simulink library "carnot"  (R2018b)
settings: Solver=VariableStepAuto  StartTime=0.0  StopTime=10.0  RelTol=1e-3
undefined symbols (not defined in the file or in its folder): A, A_earth, acol, Acol, ActPower1, ActPower2, ActPower3, Ad, Ad0, Ar, Au, Au0, Azimuth_Angle, B, Bd, Bd0, Br, Bu, Bu0, C, c1, c2, c3, c33, c4, c5, c6, CarnotCallbacks_Density, CarnotCallbacks_Enthalpy, CarnotCallbacks_Enthalpy2Temperature, CarnotCallbacks_Entropy, CarnotCallbacks_Evaporation_Enthalpy, CarnotCallbacks_GlobalMessageLevel, CarnotCallbacks_Grashof, CarnotCallbacks_Heat_Capacity, CarnotCallbacks_Kinematic_Viscosity, CarnotCallbacks_PMV_PPD, CarnotCallbacks_Prandtl, CarnotCallbacks_Saturation_Property, CarnotCallbacks_Saturation_Temperature, CarnotCallbacks_Saturation_Value_Water, CarnotCallbacks_Specific_Volume, CarnotCallbacks_Thermal_Conductivity, CarnotCallbacks_Vapour_Content, CarnotCallbacks_Vapour_Pressure, Cd, Cdl, Cr, Cu, Davies, Dd, DE_TRY2010_04_averageYear, delta_grd, density, DiameterLastPiece, dl, DPConstant, DPLinear, DPQuadratic, Dr ... (+59)
libraries: $bdroot x429, simulink x36, simulink_extras x12
(part 10 of 22)

== system carnot/Source/Solar_Thermal ==
  Collector_1xN : Subsystem  mask(collector 1xN){acol=2.3, len=2, eta0=0.8, u1=3.5, u2=0.02, u3=0, uwind=0, c_col=1e4, lin=10, qua=10, tini=20, nodes=5}
      mask prompts: acol "collector surface (aperture) in [m²]"; len "length between inlet and outlet [m]"; eta0 "optical efficiency [-]"; u1 "linear heat loss coefficient [W/(m²*K)]"; u2 "quadratic heat loss coefficient [W/(m*K)²]"; u3 "radiative loss coefficient [W/(m²*K)]"; uwind "wind dependent heat loss [W/(m²*K*m/s)]"; c_col "effective heat capacity of collector [J/(m²*K)]"; lin "linear pressure drop Pa/(kg/s)"; qua "quadratic  pressure drop Pa/(kg/s)²"; tini "initial temperature [degree Celsius]"; nodes "number of nodes"
      mask help:
      | Model for tested collectors. Enter test results in this mask.
      | Look under mask to change the incidence angle modifier, the pressure drop and the radiation calculation method.
      mask init:
      | acol = max(acol, 0.01);
      | eta0 = max(eta0,0);
      | c_col = max(c_col, 0.1);
      mask Help: web(fullfile(path_carnot('help'),'Collector_1xN.html'),'-helpbrowser')
      mask DialogControl ParameterTabVar0 Prompt: Geometry
      mask DialogControl ParameterTabVar01 Prompt: Coll.Parameters
      mask DialogControl ParameterTabVar012 Prompt: Hydraulic
      mask DialogControl ParameterTabVar0123 Prompt: Calculation
      mask Display: plot(-10,0,80,78,[10 16 66 60 10],[16 10 60 66 16],[8,13],[8,13],[63,68],[63,68])
  Collector_Unglazed : Subsystem  mask(Unglazed solar thermal collector){tini=0.1, Ncollector=1, PathName=fullfile(path_carnot('libsl'), 'Source', 'Solar_Thermal', 'Collector_Unglazed', 'parameter_set'), FileName='DefaultCollectorUnglazed.mat', userPath=off, userParam=off, acol=2.544, len=2.1, nodes=10, fta=0.9, eps=0.9, u0l=40, u0c=1, u0g=40, u1l=8, u1c=1, u1g=8, u1e=0.01, hi=200, capa=5000, capf=4000, SensorTimeConstant=10, dplin=5504.4, dpqua=6222.096}
      mask prompts: tini "Initial temperature [°C]"; Ncollector "Number of collectors in parallel"; PathName "Path"; FileName "Parameter set"; userPath "Edit path and name of parameter set"; userParam "User defined parameters"; acol "Collector surface (aperture) in [m²]"; len "Length between inlet and outlet [m]"; nodes "Number of nodes (>=2)"; fta "Absorption coefficient of the absorber [-]"; eps "Thermal emissivity of the absorber (0..1)"; u0l "U0L heat transfer for losses [W/(m²*K)]"; u0c "U0C heat transfer for condensation [W/(m²*K)]"; u0g "U0G heat transfer for gains [W/(m²*K)]"; u1l "U1L wind dependent heat transfer for losses [W/(m²*K*m/s)]"; u1c "U1C wind dependent heat transfer for condensation [W/(m²*K*m/s)]"; u1g "U1G wind dependent heat transfer for gains [W/(m²*K*m/s)]"; u1e "U1E wind dependancy of optical efficiency in W/(m²*m/s)"; hi "HI heat transfer between collector and tube [W/(m²*K)]"; capa "Effective heat capacity of absorber [J/(m²*K)]"; capf "Effective heat capacity of fluid [J/(m²*K)]"; SensorTimeConstant "Time constant of temperature sensor [s]"; dplin "Linear pressure drop in Pa/(kg/s)"; dpqua "Quadratic pressure drop in Pa/(kg/s)²"
      mask help:
      | 2xN node model for an unglazed solar thermal collectors including condensation effects for temperatures below dewpoint.
      | c_abs*dTp/dt=qdot_solar-qdot_conv_gain-qdot_conv_loss-qdot_cond -qdot_sky-qdot_fluid
      | qdot_solar = absorbed_solar_radiation - U1E*Iglb*vwind
      | qdot_conv_gain = fconv * (U0G + U1G*vwind)*(Tp - Tamb)
      | qdot_conv_loss = (1-fconv)*(U0L + U1L*vwind)*(Tp - Tamb)
      | qdot_cond = fcond*(U0C + U1C*vwind)*ccond*(ps(Tdew) - ps(Tp))
      | qdot_sky = e * const_sigma*((Tp+273)^4 - (Tsky+273)^4)
      | qdot_fluid = HI*(Tp-Tfluid)
      | fconv = 1 if Tp > Tamb, 0 otherwise
      | fcond = 1 if Tp below dewpoint, 0 otherwise
      mask init:
      | [ok, param] = CarnotCallbacks_CollectorUnglazedConf('SetParameters',gcbh,PathName,FileName);
      mask Help: web(fullfile(path_carnot('help'),'Collector_Unglazed.html'),'-helpbrowser')
      mask TypeOptions tini: Collector_Unglazed/tini | T_Sensor1/t0
      mask TypeOptions Ncollector: Ncollector/Value | Gain/Gain | Gain3/Gain
      mask Callback userPath: [ok, param] = CarnotCallbacks_CollectorUnglazedConf('UserEdit',gcbh);
      mask Callback userParam: [ok, param] = CarnotCallbacks_CollectorUnglazedConf('UserEdit',gcbh);
      mask TypeOptions acol: Collector_Unglazed/acol
      mask TypeOptions len: Collector_Unglazed/len
      mask TypeOptions nodes: Collector_Unglazed/nodes
      mask TypeOptions fta: Collector_Unglazed/fta
      mask TypeOptions eps: Collector_Unglazed/e_sky
      mask TypeOptions u0l: Collector_Unglazed/uc0loss
      mask TypeOptions u0c: Collector_Unglazed/uc0
      mask TypeOptions u0g: Collector_Unglazed/uc0gain
      mask TypeOptions u1l: Collector_Unglazed/uc1loss
      mask TypeOptions u1c: Collector_Unglazed/uc1
      mask TypeOptions u1g: Collector_Unglazed/uc1gain
      mask TypeOptions u1e: Collector_Unglazed/uc1eta0
      mask TypeOptions hi: Collector_Unglazed/hi
      mask TypeOptions capa: Collector_Unglazed/c_abs
      mask TypeOptions capf: Collector_Unglazed/c_fl
      mask TypeOptions SensorTimeConstant: T_Sensor1/tc
      mask TypeOptions dplin: Collector_Unglazed/lin
      mask TypeOptions dpqua: Collector_Unglazed/qua
      mask DialogControl Container7 Prompt: Calculation
      mask DialogControl ParameterGroupVar Prompt: Picking a parameter set
      mask DialogControl Control3 Prompt: Carnot public data
      mask DialogControl Control3 Callback: [ok, file] = CarnotCallbacks_CollectorUnglazedConf('GetFilename',gcbh, 'public');
      mask DialogControl Control4 Prompt: Carnot internal data
      mask DialogControl Control4 Callback: [ok, file] = CarnotCallbacks_CollectorUnglazedConf('GetFilename',gcbh, 'internal');
      mask DialogControl Control2 Prompt: Selected path
      mask DialogControl Control2 Callback: [ok, file] = CarnotCallbacks_CollectorUnglazedConf('GetFilename',gcbh, 'selected');
      mask DialogControl Container9 Prompt: Parameter values
      mask DialogControl Container8 Prompt: Geometry
      mask DialogControl Container11 Prompt: Thermal
      mask DialogControl Container12 Prompt: Hydraulic
      mask DialogControl Control6 Prompt: Save in Carnot internal data
      mask DialogControl Control6 Callback: [ok, param] = CarnotCallbacks_CollectorUnglazedConf('SaveFilename',gcbh, 'internal','USTC');
      mask DialogControl Control5 Prompt: Save in selected path
      mask DialogControl Control5 Callback: [ok, param] = CarnotCallbacks_CollectorUnglazedConf('SaveFilename',gcbh, 'selected','USTC');
      mask Display:
      | % user defined picture file
      | picfile = fullfile(path_carnot('intlibsl'), ...
      |     'Source','Solar_Thermal','Collector_Unglazed','parameter_set', ...
      |      'Collector_CONF.jpg');
      | 
      | pic = false;
      | 
      | % show internal picture if defined
      | if ~BlockIsInCarnotLibrary    % if not located in library any more
      |     if exist(picfile)
      |         image(imread(picfile), [0.2, 0, 0.7, 1])
      |         set_param(gcb, 'BackgroundColor', 'White')
      |         pic = true;
      |     end
      | end
      | 
      | if ~pic % show public picture
      |     plot([0,70,70,0,0]/140+0.1,         [-0,-0,5,5,-0]/140+0.2, ...
      |         [30,30,100,100,30]/140+0.1,     [100,94,94,100,100]/140+0.2, ...
      |         [32,1]/140+0.1,                 [94,5]/140+0.2, ...
      |         [40,10]/140+0.1,                [94,5]/140+0.2, ...
      |         [49,19]/140+0.1,                [94,5]/140+0.2, ...
      |         [57,27]/140+0.1,                [94,5]/140+0.2, ...
      |         [65,35]/140+0.1,                [94,5]/140+0.2, ...
      |         [73,43]/140+0.1,                [94,5]/140+0.2, ...
      |         [82,51]/140+0.1,                [94,5]/140+0.2, ...
      |         [90,60]/140+0.1,                [94,5]/140+0.2,...
      |         [98,68]/140+0.1,                [94,5]/140+0.2)
      |     set_param(gcb, 'BackgroundColor', 'Yellow')
      | end
  Collector_Unglazed_ISO9806 : Subsystem  mask(Unglazed solar thermal collector){tini=1, Ncollector=2, PathName='current', FileName='Viessmann_SLK_ISO9806_lowCp.mat', userPath=off, userParam=off, acol=2.544, len=2.1, eta0=0.702, bu=0.066, b1=32.64, b2=3.59, c_abs=2*3900, dplin=5504.4, dpqua=6222.096}
      mask prompts: tini "Initial temperature [°C]"; Ncollector "Number of collectors in parallel"; PathName "Path"; FileName "Parameter set"; userPath "Edit path and name of parameter set"; userParam "User defined parameters"; acol "Collector surface (aperture) in [m²]"; len "Length between inlet and outlet [m]"; eta0 "Optical efficiency Eta0 [-]"; bu "bu: wind dependancy of optical efficiency in W/(m²*m/s)"; b1 "b1: heat transfer for losses [W/(m²*K)]"; b2 "b2: wind dependent heat transfer for losses [W/(m²*K*m/s)]"; c_abs "Effective heat capacity of absorber [J/(m²*K)]"; dplin "Linear pressure drop in Pa/(kg/s)"; dpqua "Quadratic pressure drop in Pa/(kg/s)²"
      mask help:
      | ISO 9806 model of an unglazed solar thermal collector.
      |  Qdot = A*G*(eta0*(1-bu*vwind) - (b1 + b2*vwind)*(Tm-Tamb)/G)
      |  Qdot = mdot*cp*(Tout-Tin)
      |  Tm = (Tout+Tin)/2
      |  Tout = 2*Tm - Tin
      |  CapAbs*dTm/dt = -mdot*cp*(Tout-Tin)/A + (G*eta0*(1-bu*vwind) - (b1 + b2*vwind)*(Tm-Tamb))
      | Keep in mind that the ISO equation is not respecting the energy conservation for variable inlet conditions (e.g. temperature).
      | IT IS RECOMMENDED TO USE THIS MODEL ONLY FOR STEADY STATE CONDITIONS AT THE INLET (use Collector_Unglazed_ISO_2node model for system simulation).
      mask init:
      | [ok, param] = CarnotCallbacks_CollectorUnglazedConf('SetParameters',gcbh,PathName,FileName);
      mask Help: web(fullfile(path_carnot('help'),'Collector_Unglazed_ISO9806.html'),'-helpbrowser')
      mask TypeOptions tini: Integrator/InitialCondition
      mask TypeOptions Ncollector: ncol/Gain | ncol1/Gain | Constant/Value
      mask Callback userPath: [ok, param] = CarnotCallbacks_CollectorUnglazedISO9806('UserEdit',gcbh);
      mask Callback userParam: [ok, param] = CarnotCallbacks_CollectorUnglazedISO9806('UserEdit',gcbh);
      mask TypeOptions acol: acol/Value | acol1/Value
      mask TypeOptions len: Pressure_Drop_Collector/len
      mask TypeOptions eta0: eta0/Gain
      mask TypeOptions bu: bu/Gain
      mask TypeOptions b1: b1/Bias
      mask TypeOptions b2: b2/Gain
      mask TypeOptions c_abs: c_abs/Value
      mask TypeOptions dplin: Pressure_Drop_Collector/lin
      mask TypeOptions dpqua: Pressure_Drop_Collector/qua
      mask DialogControl Container7 Prompt: Calculation
      mask DialogControl ParameterGroupVar Prompt: Picking a parameter set
      mask DialogControl Control3 Prompt: Carnot public data
      mask DialogControl Control3 Callback: [ok, file] = CarnotCallbacks_CollectorUnglazedISO9806('GetFilename',gcbh, 'public');
      mask DialogControl Control4 Prompt: Carnot internal data
      mask DialogControl Control4 Callback: [ok, file] = CarnotCallbacks_CollectorUnglazedISO9806('GetFilename',gcbh, 'internal');
      mask DialogControl Control2 Prompt: Selected path
      mask DialogControl Control2 Callback: [ok, file] = CarnotCallbacks_CollectorUnglazedISO9806('GetFilename',gcbh, 'selected');
      mask DialogControl Container9 Prompt: Parameter values
      mask DialogControl Container8 Prompt: Geometry
      mask DialogControl Container11 Prompt: Thermal
      mask DialogControl Container12 Prompt: Hydraulic
      mask DialogControl Control6 Prompt: Save in Carnot internal data
      mask DialogControl Control6 Callback: [ok, param] = CarnotCallbacks_CollectorUnglazedISO9806('SaveFilename',gcbh, 'internal','USTC');
      mask DialogControl Control5 Prompt: Save in selected path
      mask DialogControl Control5 Callback: [ok, param] = CarnotCallbacks_CollectorUnglazedISO9806('SaveFilename',gcbh, 'selected','USTC');
      mask Display:
      | % user defined picture file
      | picfile = fullfile(path_carnot('intlibsl'), ...
      |     'Source','Solar_Thermal','Collector_Unglazed_ISO9806','parameter_set','Collector_CONF.jpg');
      | 
      | pic = false;
      | 
      | % show internal picture if defined
      | if ~BlockIsInCarnotLibrary    % if not located in library any more
      |     if exist(picfile)
      |         image(imread(picfile), [0.2, 0, 0.6, 1])
      |         set_param(gcb, 'BackgroundColor', 'White')
      |         pic = true;
      |     end
      | end
      | 
      | if ~pic % show public picture
      |     disp('ISO 9806 unglazed\n\n\n\n\n\n\n\n\n\n')
      |     plot([0,70,70,0,0]/140+0.1,         [-0,-0,5,5,-0]/140+0.1, ...
      |         [30,30,100,100,30]/140+0.1,     [100,94,94,100,100]/140+0.1, ...
      |         [32,1]/140+0.1,                 [94,5]/140+0.1, ...
      |         [40,10]/140+0.1,                [94,5]/140+0.1, ...
      |         [49,19]/140+0.1,                [94,5]/140+0.1, ...
      |         [57,27]/140+0.1,                [94,5]/140+0.1, ...
      |         [65,35]/140+0.1,                [94,5]/140+0.1, ...
      |         [73,43]/140+0.1,                [94,5]/140+0.1, ...
      |         [82,51]/140+0.1,                [94,5]/140+0.1, ...
      |         [90,60]/140+0.1,                [94,5]/140+0.1,...
      |         [98,68]/140+0.1,                [94,5]/140+0.1)
      |     set_param(gcb, 'BackgroundColor', 'Yellow')
      | end
  Collector_Unglazed_ISO_2node : Subsystem  mask(Unglazed solar thermal collector){tini=20, Ncollector=1, PathName=fullfile(path_carnot('libsl'), 'Source', 'Solar_Thermal', 'Collector_Unglazed_ISO9806', 'parameter_set'), FileName='Viessmann_SLK_ISO9806.mat', userPath=off, userParam=off, acol=2.544, len=2.1, eta0=0.702, bu=0.066, b1=32.64, b2=3.59, c_abs=50*3900, dplin=5504.4, dpqua=6222.096}
      mask prompts: tini "Initial temperature [°C]"; Ncollector "Number of collectors in parallel"; PathName "Path"; FileName "Parameter set"; userPath "Edit path and name of parameter set"; userParam "User defined parameters"; acol "Collector surface (aperture) in [m²]"; len "Length between inlet and outlet [m]"; eta0 "Optical efficiency Eta0 [-]"; bu "bu: wind dependancy of optical efficiency in W/(m²*m/s)"; b1 "b1: heat transfer for losses [W/(m²*K)]"; b2 "b2: wind dependent heat transfer for losses [W/(m²*K*m/s)]"; c_abs "Effective heat capacity of absorber [J/(m²*K)]"; dplin "Linear pressure drop in Pa/(kg/s)"; dpqua "Quadratic pressure drop in Pa/(kg/s)²"
      mask help:
      | Modified ISO 9806 model of an unglazed solar thermal collector with 2 thermal capacity nodes. The first thermal node is at the inlet, the second node is at the oulet. Both nodes have half of the capacity of the ISO test report.
      |  Qdot = A*G*(eta0*(1-bu*vwind) - (b1 + b2*vwind)*(Tm-Tamb)/G)
      |  Qdot = mdot*cp*(Tout-Tin)
      |  Tm = (Tout+Tin)/2
      |  dTin/dt = mdot*cp*(Tinlet-Tin)*2/(Acol*Ncol*CapAbs)
      |  dTout/dt = (-mdot*cp*(Tout-Tin)/(Acol*Ncol) + (G*eta0*(1-bu*vwind) - (b1 + b2*vwind)*(Tm-Tamb)))*2/CapAbs
      | This modified equations respect energy conservation also for variable inlet conditions (e.g. temperature).
      | IT IS RECOMMENDED TO USE THIS MODEL FOR SYSTEM SIMULATIONS (instead of the Collector Unglazed ISO 9806 model).
      mask init:
      | % callback to set parameters of model
      | [ok, param] = CarnotCallbacks_CONFblocksMain('SetParameters',gcbh,PathName,FileName, ...
      |     fullfile('Source','Solar_Thermal','Collector_Unglazed_ISO_2node','parameter_set'));
      | 
      | % [ok, param] = CarnotCallbacks_CollectorUnglazedConf('SetParameters',gcbh,PathName,FileName);
      mask Help: web(fullfile(path_carnot('help'),'Collector_Unglazed_ISO_2node.html'),'-helpbrowser')
      mask TypeOptions tini: Integrator/InitialCondition | Tin_node/Integrator/InitialCondition
      mask TypeOptions Ncollector: ncol/Gain | Pressure Drop/Ncoll/Value
      mask Callback userPath:
      | [ok, param] = CarnotCallbacks_CONFblocksMain('UserEdit',gcbh,...
      |     'userPath','userParam','FileName');
      mask Callback userParam: [ok, param] = CarnotCallbacks_CONFblocksMain('UserEdit',gcbh,'userPath','userParam','FileName');
      mask TypeOptions acol: acol/Value
      mask TypeOptions len: Pressure Drop/Pressure_Drop_Collector/len
      mask TypeOptions eta0: eta0/Gain
      mask TypeOptions bu: bu/Gain
      mask TypeOptions b1: b1/Bias
      mask TypeOptions b2: b2/Gain
      mask TypeOptions c_abs: c_abs/Value
      mask TypeOptions dplin: Pressure Drop/Pressure_Drop_Collector/lin
      mask TypeOptions dpqua: Pressure Drop/Pressure_Drop_Collector/qua
      mask DialogControl Container7 Prompt: Calculation
      mask DialogControl ParameterGroupVar Prompt: Picking a parameter set
      mask DialogControl Control3 Prompt: Carnot public data
      mask DialogControl Control3 Callback:
      | [ok,file] = CarnotCallbacks_CONFblocksMain('GetFilename',gcbh, 'public', ...
      |     fullfile('Source','Solar_Thermal','Collector_Unglazed_ISO_2node','parameter_set'), ...
      |     'userPath','userParam','PathName','FileName');
      mask DialogControl Control4 Prompt: Carnot internal data
      mask DialogControl Control4 Callback:
      | [ok,file] = CarnotCallbacks_CONFblocksMain('GetFilename',gcbh, 'internal', ...
      |     fullfile('Source','Solar_Thermal','Collector_Unglazed_ISO_2node','parameter_set'), ...
      |     'userPath','userParam','PathName','FileName');
      mask DialogControl Control2 Prompt: Selected path
      mask DialogControl Control2 Callback:
      | [ok,file] = CarnotCallbacks_CONFblocksMain('GetFilename',gcbh, 'selected', ...
      |     fullfile('Source','Solar_Thermal','Collector_Unglazed_ISO_2node','parameter_set'), ...
      |     'userPath','userParam','PathName','FileName');
      mask DialogControl Container9 Prompt: Parameter values
      mask DialogControl Container8 Prompt: Geometry
      mask DialogControl Container11 Prompt: Thermal
      mask DialogControl Container12 Prompt: Hydraulic
      mask DialogControl Control6 Prompt: Save in Carnot internal data
      mask DialogControl Control6 Callback:
      | [ok, param] = CarnotCallbacks_CONFblocksMain('SaveFilename',gcbh,'internal','USTC', ...
      |     fullfile('Source','Solar_Thermal','Collector_Unglazed_ISO_2node','parameter_set'), ...
      |     'userPath','userParam','PathName','FileName');
      mask DialogControl Control5 Prompt: Save in selected path
      mask DialogControl Control5 Callback:
      | [ok, param] = CarnotCallbacks_CONFblocksMain('SaveFilename',gcbh,'selected','USTC', ...
      |     fullfile('Source','Solar_Thermal','Collector_Unglazed_ISO_2node','parameter_set'), ...
      |     'userPath','userParam','PathName','FileName');
      mask Display:
      | % user defined picture file
      | picfile = fullfile(path_carnot('intlibsl'), ...
      |     'Source','Solar_Thermal','Collector_Unglazed_ISO_2node','parameter_set','Collector_CONF.jpg');
      | 
      | pic = false;
      | 
      | % show internal picture if defined
      | if ~BlockIsInCarnotLibrary    % if not located in library any more
      |     if exist(picfile)
      |         image(imread(picfile), [0.2, 0, 0.6, 1])
      |         set_param(gcb, 'BackgroundColor', 'White')
      |         pic = true;
      |     end
      | end
      | 
      | if ~pic % show public picture
      |     disp('ISO unglazed 2 node\n\n\n\n\n\n\n\n\n\n')
      |     plot([0,70,70,0,0]/140+0.1,         [-0,-0,5,5,-0]/140+0.1, ...
      |         [30,30,100,100,30]/140+0.1,     [100,94,94,100,100]/140+0.1, ...
      |         [32,1]/140+0.1,                 [94,5]/140+0.1, ...
      |         [40,10]/140+0.1,                [94,5]/140+0.1, ...
      |         [49,19]/140+0.1,                [94,5]/140+0.1, ...
      |         [57,27]/140+0.1,                [94,5]/140+0.1, ...
      |         [65,35]/140+0.1,                [94,5]/140+0.1, ...
      |         [73,43]/140+0.1,                [94,5]/140+0.1, ...
      |         [82,51]/140+0.1,                [94,5]/140+0.1, ...
      |         [90,60]/140+0.1,                [94,5]/140+0.1,...
      |         [98,68]/140+0.1,                [94,5]/140+0.1)
      |     set_param(gcb, 'BackgroundColor', 'Yellow')
      | end
  IncidenceAngleModifier : Subsystem
  PressureDropCollector : Subsystem
  SolarCollector : Subsystem  mask(Solar Thermal Collector){t0=20, Ncollector=1, PathName=fullfile(path_carnot('libsl'), 'Source', 'Solar_Thermal', 'SolarCollector', 'parameter_set'), FileName='DefaultCollector.mat', userPath=off, userParam=off, acol=3.5, len=0.1, fta=0.7, c1=1.1, c2=0.001, c3=0, c4=0, c5=5000, c6=0, KbAngles=[0 5 10 15 20 25 30 35 40 45 50 55 60 65 70 75 80 85 90], KbL=[1 1 0.9999 0.9996 0.9991 0.9982 0.9965 0.9935 0.9886 0.9807 0.9678 0.9473 0.9148 0.8638 0.7846 0.6644 0.4907 0.2599 0], KbT=[1 1 1 1 1 1 1 1 1 1 1 0.875 0.75 0.625 0.5 0.375 0.25 0.125 0], Kd=0.92, dplin=10, dpqua=10, SensorTimeConstant=10}
      mask prompts: t0 "Initial temperature [°C]"; Ncollector "Number of collectors in parallel"; PathName "Path"; FileName "Parameter set"; userPath "Edit path and name of parameter set"; userParam "User defined parameters"; acol "A: surface  of one collector module in m²"; len "Length between collector inlet and outlet in m"; fta "Fin Efficiency * Transmission * Absorption (F'(tau alfa))"; c1 "c1 : heat loss coefficient at (Tm-Ta)=0  [W/(m²*K)]"; c2 "c2: temperature dependence of the heat loss coefficient [W/(m*K)²]"; c3 "c3 : wind speed dependence of the heat loss coefficient [J/(m³K)]"; c4 "c4 : sky temperature dependence of the heat loss coefficient [W/(m²K)]"; c5 "c5 : effective thermal capacity [J/(m²K)]"; c6 "c6 : wind dependence in the zero loss efficiency [s/m]"; KbAngles "Kb: angles for longitudinal and transversal IAM [degree]"; KbL "KbL: values for longitudinal incidence angle modifier (0..1)"; KbT "KbT: values for transversal incidence angle modifier (0..1)"; Kd "Kd : Incidence angle modifier diffuse radiation"; dplin "lin: linear pressure drop in Pa/(kg/s)"; dpqua "qua: quadratic pressure drop in Pa/(kg/s)²"; SensorTimeConstant "time constant of sensor [s]"
      mask help:
      | Model for glazed solar thermal collector according to ISO 9806 standard.
      | c5 dTm/dt = F'(TauAlfa) (Kdir Idir + Kdfu Idfu) - (Tm-Tamb) (c1 + c2 (Tm-Tamb)) - v_wind (c3 (Tm-Ta) + c6 Iglb) + c4 (ELongwave - sigma_SB Tamb^4) - mdot cp (Tout-Tin) /A
      | Tm = (Tin+Tout)/2
      | Keep in mind that the ISO equation is not respecting the energy conservation for variable inlet conditions (e.g. temperature).
      | IT IS RECOMMENDED TO USE THIS MODEL ONLY FOR STEADY STATE CONDITIONS AT THE INLET (use Collector_Unglazed_ISO_2node model for system simulation).
      mask init:
      | % callback to set parameters of model
      | [ok, param] = CarnotCallbacks_CollectorEN12975Conf('SetParameters',gcbh,PathName,FileName);
      mask Help: web(fullfile(path_carnot('help'),'collector_en12975.html'),'-helpbrowser')
      mask TypeOptions t0: T_Sensor/t0 | glazed_collector_ISO9806/tini
      mask TypeOptions Ncollector: Ncollector/Value | Gain1/Gain | Gain2/Gain
      mask Callback userPath: [ok, param] = CarnotCallbacks_CollectorEN12975Conf('UserEdit',gcbh);
      mask Callback userParam: [ok, param] = CarnotCallbacks_CollectorEN12975Conf('UserEdit',gcbh);
      mask TypeOptions acol: glazed_collector_ISO9806/acol | Acol/Value
      mask TypeOptions len: Pressure_Drop_Collector/len
      mask TypeOptions fta: glazed_collector_ISO9806/fta
      mask TypeOptions c1: glazed_collector_ISO9806/c1
      mask TypeOptions c2: glazed_collector_ISO9806/c2
      mask TypeOptions c3: glazed_collector_ISO9806/c3
      mask TypeOptions c4: glazed_collector_ISO9806/c4
      mask TypeOptions c5: glazed_collector_ISO9806/c5
      mask TypeOptions c6: glazed_collector_ISO9806/c6
      mask TypeOptions KbAngles: glazed_collector_ISO9806/kblangle | glazed_collector_ISO9806/kbtangle
      mask TypeOptions KbL: glazed_collector_ISO9806/KbL
      mask TypeOptions KbT: glazed_collector_ISO9806/KbT
      mask TypeOptions Kd: glazed_collector_ISO9806/Kd
      mask TypeOptions dplin: Pressure_Drop_Collector/lin
      mask TypeOptions dpqua: Pressure_Drop_Collector/qua
      mask TypeOptions SensorTimeConstant: T_Sensor/tc
      mask DialogControl ParameterGroupVar Prompt: Picking a parameter set
      mask DialogControl Control2 Prompt: Carnot public data
      mask DialogControl Control2 Callback: [ok, file] = CarnotCallbacks_CollectorEN12975Conf('GetFilename',gcbh,'public');
      mask DialogControl Control3 Prompt: Carnot internal data
      mask DialogControl Control3 Callback: [ok, file] = CarnotCallbacks_CollectorEN12975Conf('GetFilename',gcbh,'internal');
      mask DialogControl Control4 Prompt: Selected path
      mask DialogControl Control4 Callback: [ok, file] = CarnotCallbacks_CollectorEN12975Conf('GetFilename',gcbh,'selected');
      mask DialogControl Container7 Prompt: Geometry
      mask DialogControl Container8 Prompt: Coll.Params
      mask DialogControl Container9 Prompt: Optics
      mask DialogControl Container10 Prompt: Hydraulic
      mask DialogControl Container11 Prompt: Sensors
      mask DialogControl Control5 Prompt: Save in Carnot interal data
      mask DialogControl Control5 Callback: [ok, param] = CarnotCallbacks_CollectorEN12975Conf('SaveFilename',gcbh,'internal','COL');
      mask DialogControl Control6 Prompt: Save in seleced path
      mask DialogControl Control6 Callback: [ok, param] = CarnotCallbacks_CollectorEN12975Conf('SaveFilename',gcbh,'selected','COL');
      mask Display:
      | % user defined picture file
      | picfile = fullfile(path_carnot('intlibsl'), ...
      |     'Source','Solar_Thermal','SolarCollector','parameter_set', ...
      |      'Collector_CONF.jpg');
      | 
      | pic = false;
      | 
      | % show internal picture if defined
      | if ~BlockIsInCarnotLibrary    % if not located in library any more
      |     if exist(picfile)
      |         image(imread(picfile), [0.2, 0, 0.6, 1])
      |         set_param(gcb, 'BackgroundColor', 'White')
      |         pic = true;
      |     end
      | end
      | 
      | if ~pic    % show public picture
      |     disp('Solar Thermal\nCollector\n\nISO 9806')
      |     set_param(gcb, 'BackgroundColor', 'Yellow')
      | end
  SolarCollector_2node : Subsystem  mask(Solar Thermal Collector){t0=20, Ncollector=1, PathName=fullfile(path_carnot('libsl'), 'Source', 'Solar_Thermal', 'SolarCollector_2node', 'parameter_set'), FileName='DefaultCollector.mat', userPath=off, userParam=off, acol=3.5, len=0.1, fta=0.7, c1=1.1, c2=0.001, c3=0, c4=0, c5=5000, c6=0, KbAngles=[0 5 10 15 20 25 30 35 40 45 50 55 60 65 70 75 80 85 90], KbL=[1 1 0.9999 0.9996 0.9991 0.9982 0.9965 0.9935 0.9886 0.9807 0.9678 0.9473 0.9148 0.8638 0.7846 0.6644 0.4907 0.2599 0], KbT=[1 1 1 1 1 1 1 1 1 1 1 0.875 0.75 0.625 0.5 0.375 0.25 0.125 0], Kd=0.92, dplin=10, dpqua=10, SensorTimeConstant=10}
      mask prompts: t0 "Initial temperature [°C]"; Ncollector "Number of collectors in parallel"; PathName "Path"; FileName "Parameter set"; userPath "Edit path and name of parameter set"; userParam "User defined parameters"; acol "A: surface  of one collector module in m²"; len "Length between collector inlet and outlet in m"; fta "Fin Efficiency * Transmission * Absorption (F'(tau alfa))"; c1 "c1 : heat loss coefficient at (Tm-Ta)=0  [W/(m²*K)]"; c2 "c2: temperature dependence of the heat loss coefficient [W/(m*K)²]"; c3 "c3 : wind speed dependence of the heat loss coefficient [J/(m³K)]"; c4 "c4 : sky temperature dependence of the heat loss coefficient [W/(m²K)]"; c5 "c5 : effective thermal capacity [J/(m²K)]"; c6 "c6 : wind dependence in the zero loss efficiency [s/m]"; KbAngles "Kb: angles for longitudinal and transversal IAM [degree]"; KbL "KbL: values for longitudinal incidence angle modifier (0..1)"; KbT "KbT: values for transversal incidence angle modifier (0..1)"; Kd "Kd : Incidence angle modifier diffuse radiation"; dplin "lin: linear pressure drop in Pa/(kg/s)"; dpqua "qua: quadratic pressure drop in Pa/(kg/s)²"; SensorTimeConstant "time constant of sensor [s]"
      mask help:
      | Modified ISO 9806 model for a glazed solar thermal collector with 2 thermal capacity nodes. The first thermal node is at the inlet, the second node is at the oulet. Both nodes have half of the capacity of the ISO test report.
      |  dTin/dt = mdot*cp*(Tinlet-Tin)*2/(Acol*Ncol*CapAbs)
      |  c5/2 dTout/dt = F'(TauAlfa) (Kdir Idir + Kdfu Idfu) - (Tm-Tamb) (c1 + c2 (Tm-Tamb))
      |                               - v_wind (c3 (Tm-Ta) + c6 Iglb) + c4 (ELongwave - sigma_SB Tamb^4)
      |                               - mdot cp (Tout-Tin) /Acol
      | This modified equations respect energy conservation also for variable inlet conditions (e.g. temperature).
      | IT IS RECOMMENDED TO USE THIS MODEL FOR SYSTEM SIMULATIONS (instead of the ISO 9806 SolarCollector model).
      mask init:
      | % callback to set parameters of model
      | [ok, param] = CarnotCallbacks_CollectorEN12975Conf('SetParameters',gcbh,PathName,FileName);
      mask Help: web(fullfile(path_carnot('help'),'collector_iso_2node.html'),'-helpbrowser')
      mask TypeOptions t0: T_Sensor/t0 | glazed_collector_ISO9806/tini
      mask TypeOptions Ncollector: Ncollector/Value | Gain1/Gain | Gain2/Gain
      mask Callback userPath:
      | [ok, param] = CarnotCallbacks_CONFblocksMain('UserEdit',gcbh,...
      |     'userPath','userParam','FileName');
      mask Callback userParam: [ok, param] = CarnotCallbacks_CONFblocksMain('UserEdit',gcbh,'userPath','userParam','FileName');
      mask TypeOptions acol: glazed_collector_ISO9806/acol | Acol/Value
      mask TypeOptions len: Pressure_Drop_Collector/len
      mask TypeOptions fta: glazed_collector_ISO9806/fta
      mask TypeOptions c1: glazed_collector_ISO9806/c1
      mask TypeOptions c2: glazed_collector_ISO9806/c2
      mask TypeOptions c3: glazed_collector_ISO9806/c3
      mask TypeOptions c4: glazed_collector_ISO9806/c4
      mask TypeOptions c5: glazed_collector_ISO9806/c5
      mask TypeOptions c6: glazed_collector_ISO9806/c6
      mask TypeOptions KbAngles: glazed_collector_ISO9806/kblangle | glazed_collector_ISO9806/kbtangle
      mask TypeOptions KbL: glazed_collector_ISO9806/KbL
      mask TypeOptions KbT: glazed_collector_ISO9806/KbT
      mask TypeOptions Kd: glazed_collector_ISO9806/Kd
      mask TypeOptions dplin: Pressure_Drop_Collector/lin
      mask TypeOptions dpqua: Pressure_Drop_Collector/qua
      mask TypeOptions SensorTimeConstant: T_Sensor/tc
      mask DialogControl ParameterGroupVar Prompt: Picking a parameter set
      mask DialogControl Control2 Prompt: Carnot public data
      mask DialogControl Control2 Callback:
      | [ok,file] = CarnotCallbacks_CONFblocksMain('GetFilename',gcbh, 'public', ...
      |     fullfile('Source','Solar_Thermal','SolarCollector_2node','parameter_set'), ...
      |     'userPath','userParam','PathName','FileName');
      mask DialogControl Control3 Prompt: Carnot internal data
      mask DialogControl Control3 Callback:
      | [ok,file] = CarnotCallbacks_CONFblocksMain('GetFilename',gcbh, 'internal', ...
      |     fullfile('Source','Solar_Thermal','SolarCollector_2node','parameter_set'), ...
      |     'userPath','userParam','PathName','FileName');
      mask DialogControl Control4 Prompt: Selected path
      mask DialogControl Control4 Callback:
      | [ok,file] = CarnotCallbacks_CONFblocksMain('GetFilename',gcbh, 'selected', ...
      |     fullfile('Source','Solar_Thermal','SolarCollector_2node','parameter_set'), ...
      |     'userPath','userParam','PathName','FileName');
      mask DialogControl Container7 Prompt: Geometry
      mask DialogControl Container8 Prompt: Coll.Params
      mask DialogControl Container9 Prompt: Optics
      mask DialogControl Container10 Prompt: Hydraulic
      mask DialogControl Container11 Prompt: Sensors
      mask DialogControl Control5 Prompt: Save in Carnot interal data
      mask DialogControl Control5 Callback:
      | [ok, param] = CarnotCallbacks_CONFblocksMain('SaveFilename',gcbh,'internal','COL', ...
      |     fullfile('Source','Solar_Thermal','SolarCollector_2node','parameter_set'), ...
      |     'userPath','userParam','PathName','FileName');
      mask DialogControl Control6 Prompt: Save in seleced path
      mask DialogControl Control6 Callback:
      | [ok, param] = CarnotCallbacks_CONFblocksMain('SaveFilename',gcbh,'selected','COL', ...
      |     fullfile('Source','Solar_Thermal','SolarCollector_2node','parameter_set'), ...
      |     'userPath','userParam','PathName','FileName');
      mask Display:
      | % user defined picture file
      | picfile = fullfile(path_carnot('intlibsl'), ...
      |     'Source','Solar_Thermal','SolarCollector','parameter_set', ...
      |      'Collector_CONF.jpg');
      | 
      | pic = false;
      | 
      | % show internal picture if defined
      | if ~BlockIsInCarnotLibrary    % if not located in library any more
      |     if exist(picfile)
      |         image(imread(picfile), [0.2, 0, 0.6, 1])
      |         set_param(gcb, 'BackgroundColor', 'White')
      |         pic = true;
      |     end
      | end
      | 
      | if ~pic    % show public picture
      |     disp('Solar Thermal\nCollector\n\nISO 2node')
      |     set_param(gcb, 'BackgroundColor', 'Yellow')
      | end

== system carnot/Source/Ventilation ==
  Constant_AIV : Subsystem  mask(constant AIV){Tsens=20, Tcon=20, Trad=20, mw=0.012, mco=0.01, rhoair=1.2, cpair=1004, pair=100000, nair=0.5}
      mask prompts: Tsens "sensitive temperature [degree centigrade]"; Tcon "convective room temperature [degree centigrade]"; Trad "radiative room temperature [degree centigrade]"; mw "mass of water per mass of air [kgw/kga]"; mco "mass of CO2 per mass of air"; rhoair "density of air in the room [kg/m3]"; cpair "heat capacity of air in the room [J/kgK]"; pair "air pressure in the room [Pa]"; nair "air exchange rate [1/h]"
      mask help: Create a constant Air Infiltration Ventilation Vector (AIV). The AIV is used by the building model (see /Load/Houses/Room_Radiator).
  Ventilation : Subsystem  mask(Ventilation with Heat Recovery and Window){Ahabit=50, Hroom=2, vent=0.6, rec=0.6, ppmCO2=400, ppmVOC=0, alpha=10, H=1, W=1, Nwin=1}
      mask prompts: Ahabit "A: heated surface of the house in m²"; Hroom "H: height of room in m"; vent "Air exchange rate (volume of house per hour) in 1/h"; rec "Heat recovery of ventilation in 0..1"; ppmCO2 "Concentration of CO2 in ppm"; ppmVOC "Concentration of VOC in ppm"; alpha "maximal opening angle (°)"; H "height of window (m)"; W "width of window (m)"; Nwin "Number of windows"
      mask help:
      | Model of a mechanical ventilation system with heat recovery and a ventilation with windows.
      | The model is suitable for the simple building model (/Load/Houses/House_simpe).
      mask init:
      | rec = max(0, min(1, rec));
      mask Help: web(fullfile(path_carnot('help'),'Ventilation.html'),'-helpbrowser')
      mask TypeOptions Ahabit: Ahabit/Value
      mask TypeOptions Hroom: Hroom/Gain
      mask TypeOptions vent: air_flow_rate/Gain
      mask TypeOptions rec: heatRecovery/Value
      mask TypeOptions ppmCO2: ppmCO2/Value
      mask TypeOptions ppmVOC: ppmVOC/Value
      mask TypeOptions alpha: Window_Ventilation/alpha
      mask TypeOptions H: Window_Ventilation/H
      mask TypeOptions W: Window_Ventilation/W
      mask TypeOptions Nwin: Window_Ventilation/Nwin
      mask DialogControl Container4 Prompt: Ventilation
      mask DialogControl Container5 Prompt: Windows
      mask Display:
      | plot(0,-0.2,1.2,1.2,[0.2 0.35], [0.8 0.7])
      | plot([0.35 0.65], [0.7 0.7])
      | plot([0.65 0.8], [0.7 0.8])
      | plot([0.65 0.8], [0.76 0.8])
      | plot([0.7 0.8], [0.65 0.8])
      | 
      | plot([0.2 0.35], [0.2 0.3])
      | plot([0.35 0.65], [0.3 0.3])
      | plot([0.65 0.8], [0.3 0.2])
      | plot([0.2 0.25], [0.2 0.32])
      | plot([0.2 0.35], [0.2 0.23])
      | 
      | plot ([0.45 0.45], [0 1])
      | plot ([0.55 0.55], [0 1])
      | 
      | plot ([0.45 0.55], [0.2 0.2])
      | plot ([0.45 0.55], [0.8 0.8])
      | 
      | plot ([0.45 0.55], [0 0.2])
      | plot ([0.45 0.55], [0.8 1])
  Ventilation_AIV : Subsystem  mask(ACTIVE COMPONENT){co2=400}
      mask prompts: co2 "CO2 content of air in ppm"
      mask help:
      | This block represents the AIR VENTILATION from outdoors into a zone.
      |
      | r : rate of nominal air flow between outdoors and indoor, [0,1]
      | [S] : vector for sinks and sources.
      |
      | NOTE: Mass flows of water and CO2 are taken into consideration.
      |
      | ASSUMPTION:
      | Incoming air volume flow is identical to outgoing air volume flow.
      mask init:
      | CO2norm = co2*1e-6;
      mask Help: web(fullfile(path_carnot('help'),'Ventilation_AIV.html'),'-helpbrowser')
      mask Display:
      | plot([0.2 0.35], [0.8 0.7])
      | plot([0.35 0.65], [0.7 0.7])
      | plot([0.65 0.8], [0.7 0.8])
      | plot([0.65 0.8], [0.76 0.8])
      | plot([0.7 0.8], [0.65 0.8])
      | 
      | plot([0.2 0.35], [0.2 0.3])
      | plot([0.35 0.65], [0.3 0.3])
      | plot([0.65 0.8], [0.3 0.2])
      | plot([0.2 0.25], [0.2 0.32])
      | plot([0.2 0.35], [0.2 0.23])
      | 
      | plot ([0.45 0.45], [0 1])
      | plot ([0.55 0.55], [0 1])
      | 
      | plot ([0.45 0.55], [0.2 0.2])
      | plot ([0.45 0.55], [0.8 0.8])
      | 
      | plot ([0.45 0.55], [0 0.2])
      | plot ([0.45 0.55], [0.8 1])
  Window_Ventilation : Subsystem  mask(window ventilation){alpha=10, H=1.2, W=1, Nwin=4}
      mask prompts: alpha "maximal opening angle (°)"; H "height of window (m)"; W "width of window (m)"; Nwin "Number of windows"
      mask help: Simulates the free driven ventilation through a window with an opening angle of [0,1]* max. angle. Valid for angles between 8° and 180°. Output is the VOLUME FLOW RATE in m^3/s. Calculation based on Weber.
      mask Help: web(fullfile(path_carnot('help'),'Window_Ventilation.html'),'-helpbrowser')
      mask TypeOptions Nwin: NumberOfWindows/Gain
      mask Display:
      | plot(0,10,90,80,[20 70 70 20 20],[20 20 70 70 20],...
      |     [20 70 80 30 20],[20 20 65 65 20])

== system carnot/Storage/Electric ==
  Battery_EB : Subsystem  TreatAsAtomicUnit=on  mask(electric Battery){cap_kWh=5e6/3.6e6, eta_ch=0.9, eta_dis=0.9, cap0=1, SOC_max=1, SOC_min=0, Pmax=1000, Pmin=1000, P_standby=10}
      mask prompts: cap_kWh "Capacity in kWh"; eta_ch "Charging efficiency"; eta_dis "Discharging efficiency"; cap0 "Initial charge condition (0...1)"; SOC_max "Maximal SOC [-]"; SOC_min "Minimal SOC [-]"; Pmax "Maximal input power"; Pmin "Maximal output power"; P_standby "Standby power consumption [W]"
      mask help:
      | Electric energy storage ('rechargable battery') with inverter, based on an energy balance.
      | dE/dt = P_in * efficiency
      | The model uses a single phase connection (ActPower1 in EB_in). Separate parameters are used for charging and discharging efficiency.
      | Negative power at inport EB_in is for discharging, positive vor charging.
      | If the battery is full, the power is led to the output P_over (in BatData).
      | If the battery is emtpty, the missing power is led to the output P_under (in BatData).
      | The state output gives the state of charge in 0...1.
      mask init:
      | capa = cap_kWh*1e3*3600;
      | Pmax = abs(Pmax);
      | Pmin = abs(Pmin);
      settings: MinAlgLoopOccurrences=on
      mask Help: web(fullfile(path_carnot('help'),'Battery.html'),'-helpbrowser')
      mask Display: plot(0,-10,120,100,[70,70,60,40,30,30,40,60,70,60,40,30],[80,10,-0,-0,10,80,70,70,80,90,90,80],[44,47,54,57,54,47,44],[80,76,76,80,84,84,80])
